simulink model "integrated_energy_system"  (R2024b)
settings: Solver=FixedStepDiscrete  StartTime=0.0  StopTime=1  FixedStep=1e-4  RelTol=1e-3
settings Model: Creator=sesa504213  LastModifiedBy=sesa504213

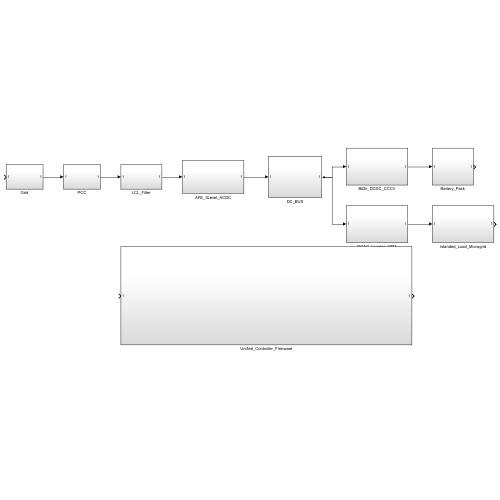
[thumbnail: Simulink's stored preview of the top-level diagram]
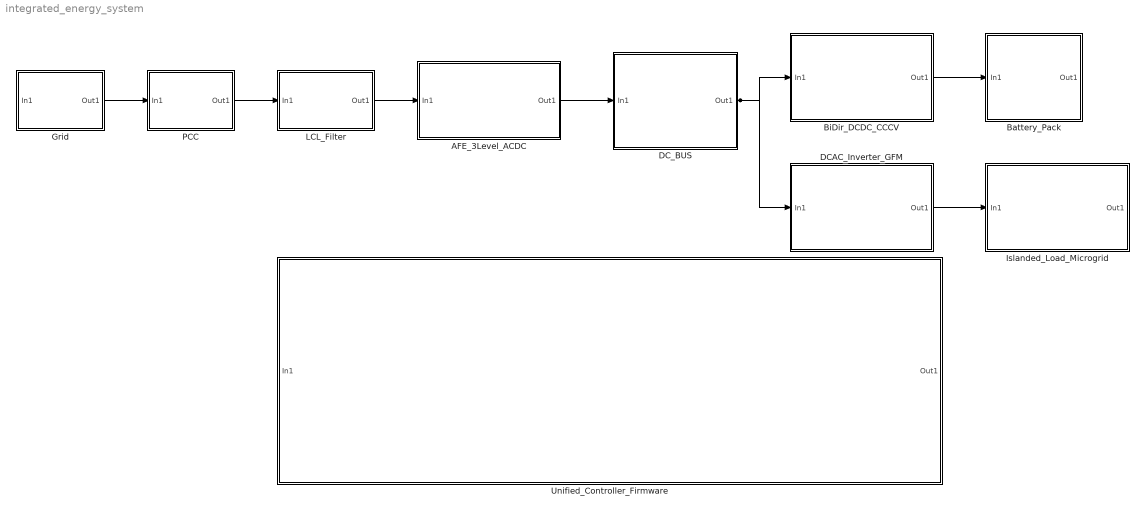
== system integrated_energy_system ==
  AFE_3Level_ACDC : Subsystem
  Battery_Pack : Subsystem
  BiDir_DCDC_CCCV : Subsystem
  DCAC_Inverter_GFM : Subsystem
  DC_BUS : Subsystem
  Grid : Subsystem
  Islanded_Load_Microgrid : Subsystem
  LCL_Filter : Subsystem
  PCC : Subsystem
  Unified_Controller_Firmware : Subsystem
  wires:
  Grid/1(Out1) -> PCC/1(In1)
  PCC/1(Out1) -> LCL_Filter/1(In1)
  LCL_Filter/1(Out1) -> AFE_3Level_ACDC/1(In1)
  AFE_3Level_ACDC/1(Out1) -> DC_BUS/1(In1)
  DC_BUS/1(Out1) -> BiDir_DCDC_CCCV/1(In1), DCAC_Inverter_GFM/1(In1)
  BiDir_DCDC_CCCV/1(Out1) -> Battery_Pack/1(In1)
  DCAC_Inverter_GFM/1(Out1) -> Islanded_Load_Microgrid/1(In1)

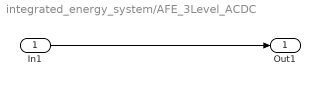
== system integrated_energy_system/AFE_3Level_ACDC ==
  In1 : Inport
  Out1 : Outport
  wires:
  In1/1 -> Out1/1

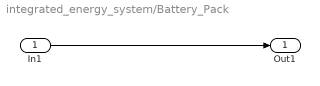
== system integrated_energy_system/Battery_Pack ==
  In1 : Inport
  Out1 : Outport
  wires:
  In1/1 -> Out1/1

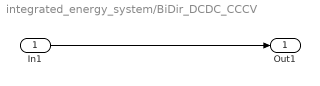
== system integrated_energy_system/BiDir_DCDC_CCCV ==
  In1 : Inport
  Out1 : Outport
  wires:
  In1/1 -> Out1/1

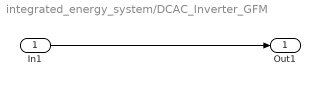
== system integrated_energy_system/DCAC_Inverter_GFM ==
  In1 : Inport
  Out1 : Outport
  wires:
  In1/1 -> Out1/1

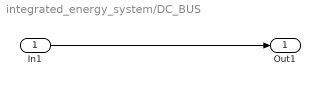
== system integrated_energy_system/DC_BUS ==
  In1 : Inport
  Out1 : Outport
  wires:
  In1/1 -> Out1/1

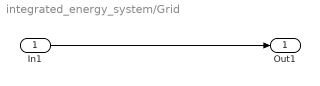
== system integrated_energy_system/Grid ==
  In1 : Inport
  Out1 : Outport
  wires:
  In1/1 -> Out1/1

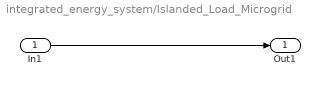
== system integrated_energy_system/Islanded_Load_Microgrid ==
  In1 : Inport
  Out1 : Outport
  wires:
  In1/1 -> Out1/1

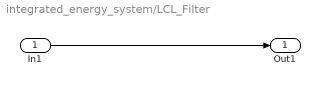
== system integrated_energy_system/LCL_Filter ==
  In1 : Inport
  Out1 : Outport
  wires:
  In1/1 -> Out1/1

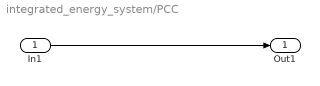
== system integrated_energy_system/PCC ==
  In1 : Inport
  Out1 : Outport
  wires:
  In1/1 -> Out1/1

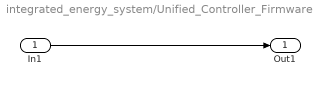
== system integrated_energy_system/Unified_Controller_Firmware ==
  In1 : Inport
  Out1 : Outport
  wires:
  In1/1 -> Out1/1
